simulink model "levitatore_function2"  (R2017a)
settings: Solver=VariableStepAuto  StartTime=0.0  StopTime=30  RelTol=1e-3
values from neighbouring files (symbols this model uses):
  par = [m,km,R,L0,b,g]    [levitatoreMagnetico.m]    (also in temp1.mat = [0.2 19.62 50 0.5 0.1 9.81])
  ueq = 5    [levitatoreMagnetico.m]    (also in temp1.mat)
  xeq = [ueq/R*sqrt(km/m/g) 0 ueq/R]    [levitatoreMagnetico.m]    (also in temp1.mat = [0.316227766017 0 0.1])
libraries: cstblocks x1
settings Model: Creator=Enrico Donato  LastModifiedBy=Enrico Donato

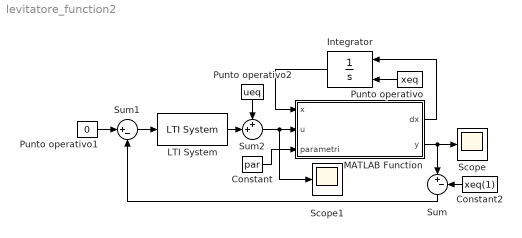
== system levitatore_function2 ==
  Constant : Constant  Value=par
  Constant2 : Constant  Value=xeq(1)
  Integrator : Integrator  InitialConditionSource=external  InitialCondition=zeros(3,1)
  LTI System : cstblocks/LTI System  sys=C2  IC=[]
  MATLAB Function : MATLAB Function  TreatAsAtomicUnit=on
  Punto operativo : Constant  Value=xeq
  Punto operativo1 : Constant  Value=0
  Punto operativo2 : Constant  Value=ueq
  Scope : Scope
  Scope1 : Scope
  Sum : Sum  Inputs=|+-
  Sum1 : Sum  Inputs=|+-
  Sum2 : Sum  Inputs=++|
  wires:
  Constant/1 -> MATLAB Function/3(parametri)
  MATLAB Function/1(dx) -> Integrator/1
  Integrator/1 -> MATLAB Function/1(x)
  MATLAB Function/2(y) -> Sum/1, Scope/1
  Punto operativo/1 -> Integrator/2
  Constant2/1 -> Sum/2
  Punto operativo1/1 -> Sum1/1
  Sum/1 -> Sum1/2
  Sum1/1 -> LTI System/1
  Sum2/1 -> MATLAB Function/2(u), Scope1/1
  Punto operativo2/1 -> Sum2/1
  LTI System/1 -> Sum2/2

== matlab function levitatore_function2/MATLAB Function ==
  data: x input; dx output; u input; y output; parametri input
function [dx,y] = fcn(x,u,parametri)
% Estrai i parametri dal terzo argomento della funzione.
m = parametri(1);
km = parametri(2);
R = parametri(3);
L = parametri(4);
b = parametri(5);
g = parametri(6);

% Definisci gli stati del modello (p,v,i).
p = x(1); v = x(2); i = x(3);

% Implementa la funzione generatrice f(x,u).
dp = v;
dv = g - (km/m)*(i/p)^2 - (b/m)*v^2;
di = (1/(L+(km/p)))*(-R*i + km*v*i/p^2 + u);

% Associa i valori alle uscite.
dx = [dp; dv; di];
y = p;
end
